simulink model "p5p3d"  (Simulink 8.9)
settings: Solver=ode45  StartTime=0.0  StopTime=1000  RelTol=1e-3  EnableMultiTasking=on
values from neighbouring files (symbols this model uses):
  course_angle = 30    [p5p3b.m]    (also in p5p3c.m; p5p3d.m)
  course_angle_error = 35    [p5p3b.m]    (also in p5p3c.m; p5p3d.m)
  K_pd = sqrt(T_f^2 * w_c^4 + w_c^2)/K    [p5p3b.m]    (also in p5p3c.m; p5p3d.m)
  T_d = T    [p5p3b.m]    (also in p5p3c.m; p5p3d.m)
  T_f = -1/(w_c* tan((180-phase_margin)*deg2rad))    [p5p3b.m]    (also in p5p3c.m; p5p3d.m)
libraries: simulink x2
settings Model: Creator=markh  LastModifiedBy=pamarton
settings DataIOCC: SignalLoggingName=sigsOut
settings OptimizationCC: InitFltsAndDblsToZero=on
settings DebuggingCC: SaveWithParameterizedLinksMsg=none  SignalResolutionControl=TryResolveAllWithWarning  MultiTaskDSMMsg=warning  MultiTaskCondExecSysMsg=none
settings HardwareCC: TargetUnknown=on
settings GRTTargetCC: TargetFcnLib=ansi_tfl_tmw.mat

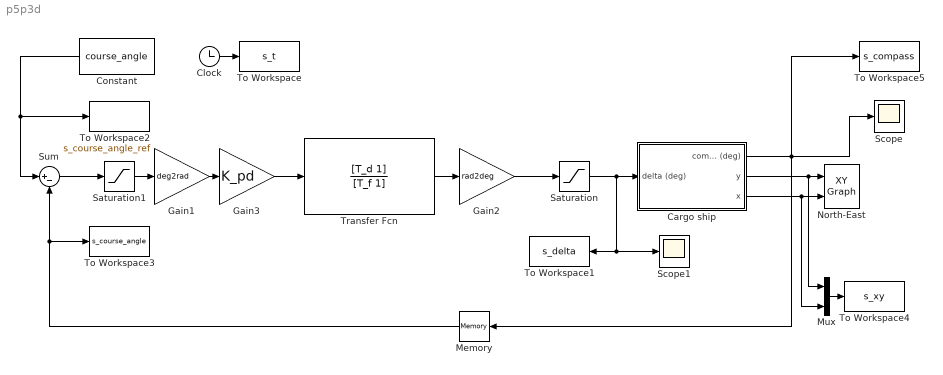
== system p5p3d ==
  Cargo ship : Subsystem  mask(Simple shipmodel for a cargo ship){noise=on, current=off, logic=on}
      mask prompts: noise "measurement noise"; logic "waves"
      mask help:
      | Measurement noise:
      | 	checked = noise on
      | 	unchecked = noise off
      |
      | Current:
      | 	checked = current on
      | 	unchecked = current off
      |
      | Waves:
      | 	checked = waves on
      | 	unchecked = waves off
      |
      | Author: Jørgen Spjøtvold, 9/10-2003
      | TTK 4115 Linear system theory.
      | Modified by Jostein Bakkeheim 26/10-2006
  Clock : Clock
  Constant : Constant  Value=course_angle
  Gain1 : Gain  Gain=deg2rad
  Gain2 : Gain  Gain=rad2deg
  Gain3 : Gain  Gain=K_pd
  Memory : Memory
  Mux : Mux  Inputs=2
  North-East : simulink/Sinks/XY Graph  xmin=-5000  xmax=5000  ymin=-5000  ymax=5000  st=-1
  Saturation : Saturate  UpperLimit=45  LowerLimit=-45
  Saturation1 : Saturate  UpperLimit=course_angle + course_angle_error  LowerLimit=course_angle - course_angle_error
  Scope : Scope
  Scope1 : Scope
  Sum : Sum  Inputs=|+-
  To Workspace : ToWorkspace  VariableName=s_t  SampleTime=-1
  To Workspace1 : ToWorkspace  VariableName=s_delta  SampleTime=-1
  To Workspace2 : ToWorkspace  VariableName=s_course_angle_ref  SampleTime=-1
  To Workspace3 : ToWorkspace  VariableName=s_course_angle  SampleTime=-1
  To Workspace4 : ToWorkspace  VariableName=s_xy  SampleTime=-1
  To Workspace5 : ToWorkspace  VariableName=s_compass  SampleTime=-1
  Transfer Fcn : TransferFcn  Numerator=[T_d 1]  Denominator=[T_f 1]
  wires:
  Cargo ship/3(x) -> Mux/2, North-East/2
  Cargo ship/1(compass (deg)) -> To Workspace5/1, Memory/1, Scope/1
  Constant/1 -> To Workspace2/1, Sum/1
  Gain2/1 -> Saturation/1
  Saturation/1 -> To Workspace1/1, Scope1/1, Cargo ship/1(delta (deg))
  Gain1/1 -> Gain3/1
  Memory/1 -> To Workspace3/1, Sum/2
  Gain3/1 -> Transfer Fcn/1
  Transfer Fcn/1 -> Gain2/1
  Saturation1/1 -> Gain1/1
  Sum/1 -> Saturation1/1
  Clock/1 -> To Workspace/1
  Cargo ship/2(y) -> Mux/1, North-East/1
  Mux/1 -> To Workspace4/1

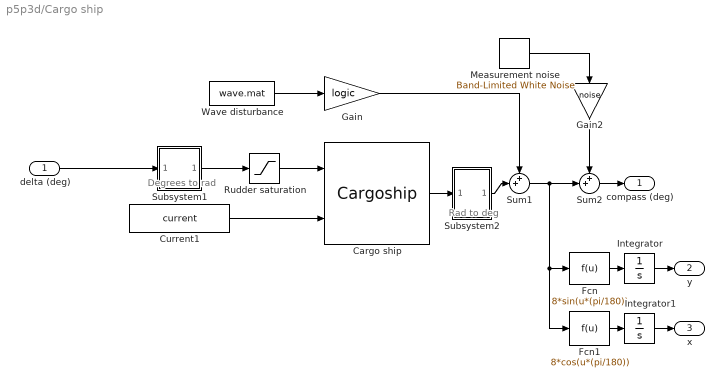
== system p5p3d/Cargo ship ==
  note: Degrees to rad
  note: Rad to deg
  delta (deg) : Inport
  Cargo ship : S-Function  FunctionName=Cargoship  SFunctionDeploymentMode=off  EnableBusSupport=off  mask(Cargo ship){}
      mask help:
      | S-function which simulates a cargo ship.
      |
      | Author: Jørgen Spjøtvold
      | 20.10-2003
      | Modified by Jostein Bakkeheim 27.10.2006
  Current1 : Constant  Value=current
  Fcn : Fcn  Expr=8*sin(u*(pi/180))
  Fcn1 : Fcn  Expr=8*cos(u*(pi/180))
  Gain : Gain  Gain=logic  SaturateOnIntegerOverflow=on  OutDataTypeStr=Inherit: Same as input  ParamDataTypeStr=Inherit: Same as input
  Gain2 : Gain  Gain=noise  SaturateOnIntegerOverflow=on  OutDataTypeStr=Inherit: Same as input  ParamDataTypeStr=Inherit: Same as input
  Integrator : Integrator
  Integrator1 : Integrator
  Measurement noise : simulink/Sources/Band-Limited White Noise  Cov=[0.001]  Ts=.5  seed=[23341]
  Rudder saturation : Saturate  UpperLimit=45*(pi/180)  LowerLimit=-45*(pi/180)
  Subsystem1 : Subsystem  mask(degrees to radians){}
      mask help: Converts degrees to radians
      mask Display: fprintf('D2R');
  Subsystem2 : Subsystem  mask(radians to degrees){}
      mask help: Converts radians to degrees
      mask Display: fprintf('R2D');
  Sum1 : Sum  Inputs=++|  SaturateOnIntegerOverflow=on
  Sum2 : Sum  Inputs=++|  SaturateOnIntegerOverflow=on
  Wave disturbance : FromFile  FileName=wave.mat  SampleTime=0
  compass (deg) : Outport
  y : Outport  Port=2
  x : Outport  Port=3
  wires:
  delta (deg)/1 -> Subsystem1/1(In1)
  Fcn/1 -> Integrator/1
  Integrator/1 -> y/1
  Fcn1/1 -> Integrator1/1
  Integrator1/1 -> x/1
  Wave disturbance/1 -> Gain/1
  Subsystem2/1(Out1) -> Sum1/2
  Gain/1 -> Sum1/1
  Sum1/1 -> Fcn/1, Fcn1/1, Sum2/2
  Cargo ship/1 -> Subsystem2/1(In1)
  Subsystem1/1(Out1) -> Rudder saturation/1
  Rudder saturation/1 -> Cargo ship/1
  Sum2/1 -> compass (deg)/1
  Measurement noise/1 -> Gain2/1
  Gain2/1 -> Sum2/1
  Current1/1 -> Cargo ship/2

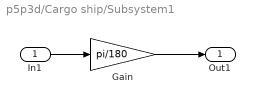
== system p5p3d/Cargo ship/Subsystem1 ==
  In1 : Inport
  Gain : Gain  Gain=pi/180  SaturateOnIntegerOverflow=on  OutDataTypeStr=Inherit: Same as input  ParamDataTypeStr=Inherit: Same as input
  Out1 : Outport
  wires:
  Gain/1 -> Out1/1
  In1/1 -> Gain/1

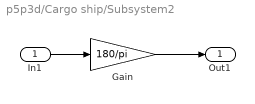
== system p5p3d/Cargo ship/Subsystem2 ==
  In1 : Inport
  Gain : Gain  Gain=180/pi  SaturateOnIntegerOverflow=on  OutDataTypeStr=Inherit: Same as input  ParamDataTypeStr=Inherit: Same as input
  Out1 : Outport
  wires:
  Gain/1 -> Out1/1
  In1/1 -> Gain/1
